simulink model "trajectory"  (R2017a)
settings: Solver=ode3  StartTime=0.0  StopTime=200  FixedStep=0.01  MaxStep=0.01  RelTol=1e-3
libraries: simulink x1
settings Model: Creator=alanik99  LastModifiedBy=Alex

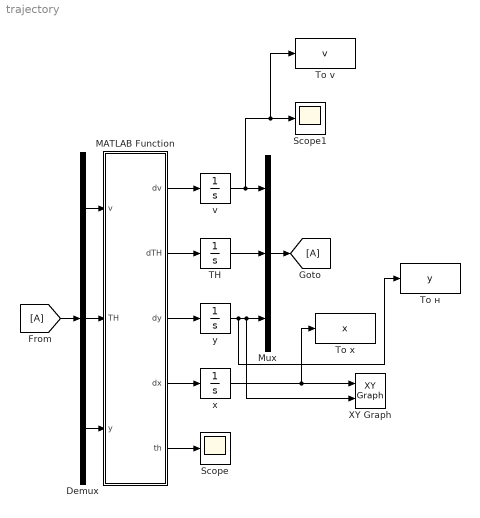
== system trajectory ==
  Demux : Demux  Outputs=3
  MATLAB Function : MATLAB Function  TreatAsAtomicUnit=on
  Mux : Mux  Inputs=3
  Scope : Scope
  Scope1 : Scope
  TH : Integrator
  To v : ToWorkspace  VariableName=v  SaveFormat=Timeseries  SampleTime=-1
  To x : ToWorkspace  VariableName=x  SaveFormat=Timeseries  SampleTime=-1
  To н : ToWorkspace  VariableName=y  SaveFormat=Timeseries  SampleTime=-1
  XY Graph : simulink/Sinks/XY Graph  xmin=0  xmax=25000  ymin=0  ymax=8000  st=-1
  v : Integrator  InitialCondition=159.44
  x : Integrator
  y : Integrator  InitialCondition=3800
  wires:
  [A] -> Demux/1
  Demux/1 -> MATLAB Function/1(v)
  MATLAB Function/1(dv) -> v/1
  Demux/3 -> MATLAB Function/3(y)
  v/1 -> To v/1, Scope1/1, Mux/1
  Mux/1 -> [A]
  Demux/2 -> MATLAB Function/2(TH)
  MATLAB Function/2(dTH) -> TH/1
  MATLAB Function/3(dy) -> y/1
  TH/1 -> Mux/2
  y/1 -> To н/1, XY Graph/2, Mux/3
  MATLAB Function/4(dx) -> x/1
  x/1 -> To x/1, XY Graph/1
  MATLAB Function/5(th) -> Scope/1

== matlab function trajectory/MATLAB Function ==
  data: dv output; dTH output; dy output; dx output; th output; v input; TH input; y input
function [dv, dTH, dy, dx, th] = fcn(v, TH, y)

m = 4000;
R = 9000;

v_i = [111.11 159.44 205.56];
Cx_i = [0.090 0.092 0.096];
Cy_i = [0.147 0.149 0.151];

if v < v_i(1) || v > v_i(end)
    
    Cx = interp1(v_i, Cx_i, v, 'linear', 'extrap');
    Cy = interp1(v_i, Cy_i, v, 'linear', 'extrap');
   
else
    Cx = interp1(v_i, Cx_i, v, 'linear');
    Cy = interp1(v_i, Cy_i, v, 'linear');
    
end

S = 16.1;
ro = 1.22*exp(-y/10000);
q = (ro * v^2) / 2;

X = Cx * q * S;
Y = Cy * q * S;

g = 9.81;
G = m*g;
a = 3;

dv = (R - X - G*sin(TH)) / m;
dTH = (R*a - G*cos(TH) + Y) / m / v;
dx = v*cos(TH);
dy = v*sin(TH);
th = TH + a;
